simulink model "phase_shift_frequency_control"  (R2018a)
settings: Solver=FixedStepDiscrete  StartTime=0.0  StopTime=stopTime  FixedStep=sampleTime  RelTol=1e-3
InitFcn:
  | fs=160e3; %Hz
  | stopTime=0.01;
  | sampleTime=1e-8;
  | deadtime= round(((1/fs)/20)/sampleTime);
  | Vdc=100;
  | Lp=82e-6;
  | Cp=1/ (Lp*4*pi*pi*150e3*150e3);
  | Rp=0.3;
  | RLOAD=10
libraries: powerlib x10
settings Model: Creator=enes_  LastModifiedBy=enes_

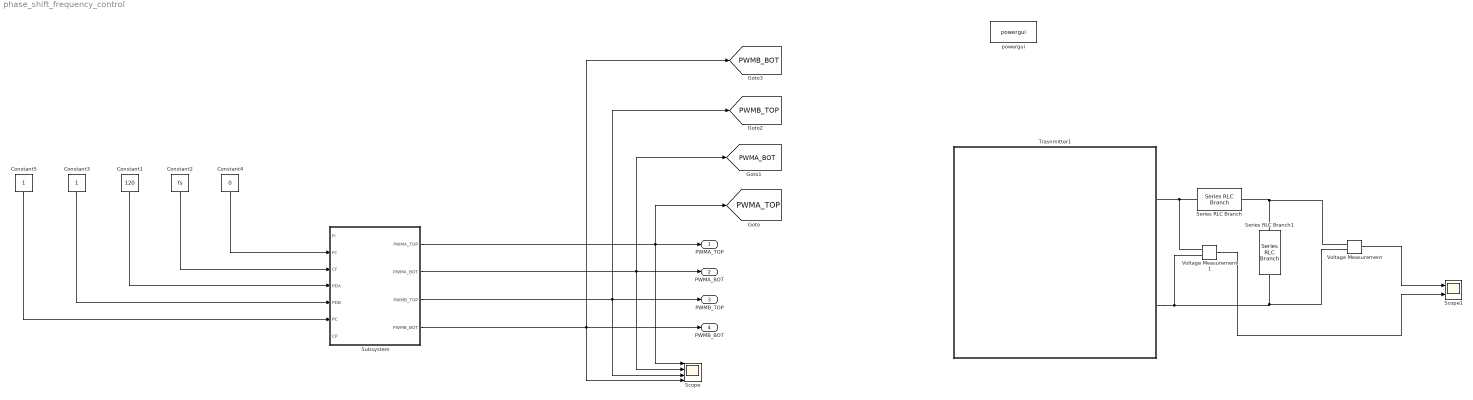
== system phase_shift_frequency_control ==
  Constant1 : Constant  Value=120
  Constant2 : Constant  Value=fs
  Constant3 : Constant
  Constant4 : Constant  Value=0
  Constant5 : Constant
  Scope : Scope  NumInputPorts=4
  Scope1 : Scope  NumInputPorts=2
  Series RLC Branch : powerlib/Elements/Series RLC Branch  LConnTagsString=__new0  RConnTagsString=__new0  BranchType=RLC  Resistance=Rp  Inductance=Lp  SetiL0=off  InitialCurrent=0  Capacitance=Cp  Setx0=off  InitialVoltage=0  Measurements=None
  Series RLC Branch1 : powerlib/Elements/Series RLC Branch  LConnTagsString=__new0  RConnTagsString=__new0  BranchType=R  Resistance=RLOAD  Inductance=Lp  SetiL0=off  InitialCurrent=0  Capacitance=Cp  Setx0=off  InitialVoltage=0  Measurements=None
  Subsystem : Subsystem
  Trasnmitter1 : Subsystem
  Voltage Measurement : powerlib/Measurements/Voltage Measurement  PhasorSimulation=off  OutputType=Complex  PSBequivalent=0
  Voltage Measurement1 : powerlib/Measurements/Voltage Measurement  PhasorSimulation=off  OutputType=Complex  PSBequivalent=0
  powergui : powerlib/powergui  Priority=1  SimulationMode=Discrete  SampleTime=sampleTime  frequency=60  Iterations=50  frequencyindice=0  Pbase=100e6  ErrMax=1e-4  UnitsV=kV  UnitsW=MW  buscounter=0  FunctionMessages=off  echomessages=off  EnableUseOfTLC=off  CurrentSourceSwitches=off  DisableSnubberDevices=off  DisableRonSwitches=off  DisableVfSwitches=off  DisplayEquations=off  SolverType=Tustin/Backward Euler (TBE)  Interpol=off  ExternalGateDelay=off  methode=off  Ts=100  x0status=blocks  SPID=on  SwTol=0  HookPort=off  RestoreLinks=warning  ResistiveCurrentMeasurement=off  Frange=[0:2:500]  Ylog=off  Xlog=on  ShowGrid=off  save=off  variable=ZData  structure=0  ZoomFFT=off  StartTime=0.0  cycles=1  DisplayStyle=1  fundamental=60  FreqAxis=off  MaxFrequency=1000  frequencyindicesteady=1  RmsSteady=1  display=off
  PWMA_TOP : Outport
  PWMA_BOT : Outport  Port=2
  PWMB_TOP : Outport  Port=3
  PWMB_BOT : Outport  Port=4
  tag scope: PWMA_BOT=global, PWMA_TOP=global, PWMB_BOT=global, PWMB_TOP=global
  wires:
  Constant4/1 -> Subsystem/2(FC)
  Constant2/1 -> Subsystem/3(CF)
  Constant1/1 -> Subsystem/4(PDA)
  Constant3/1 -> Subsystem/5(PDB)
  Constant5/1 -> Subsystem/6(PC)
  Subsystem/2(PWMA_BOT) -> [PWMA_BOT], PWMA_BOT/1, Scope/2
  Subsystem/3(PWMB_TOP) -> [PWMB_TOP], Scope/3, PWMB_TOP/1
  Subsystem/4(PWMB_BOT) -> [PWMB_BOT], Scope/4, PWMB_BOT/1
  Subsystem/1(PWMA_TOP) -> [PWMA_TOP], Scope/1, PWMA_TOP/1
  Voltage Measurement/1 -> Scope1/1
  Voltage Measurement1/1 -> Scope1/2
  connections:
  Series RLC Branch/LConn1 -- Voltage Measurement1/LConn1 -- Trasnmitter1/LConn1
  Trasnmitter1/LConn2 -- Voltage Measurement1/LConn2 -- Voltage Measurement/LConn2 -- Series RLC Branch1/RConn1
  Series RLC Branch1/LConn1 -- Voltage Measurement/LConn1 -- Series RLC Branch/RConn1

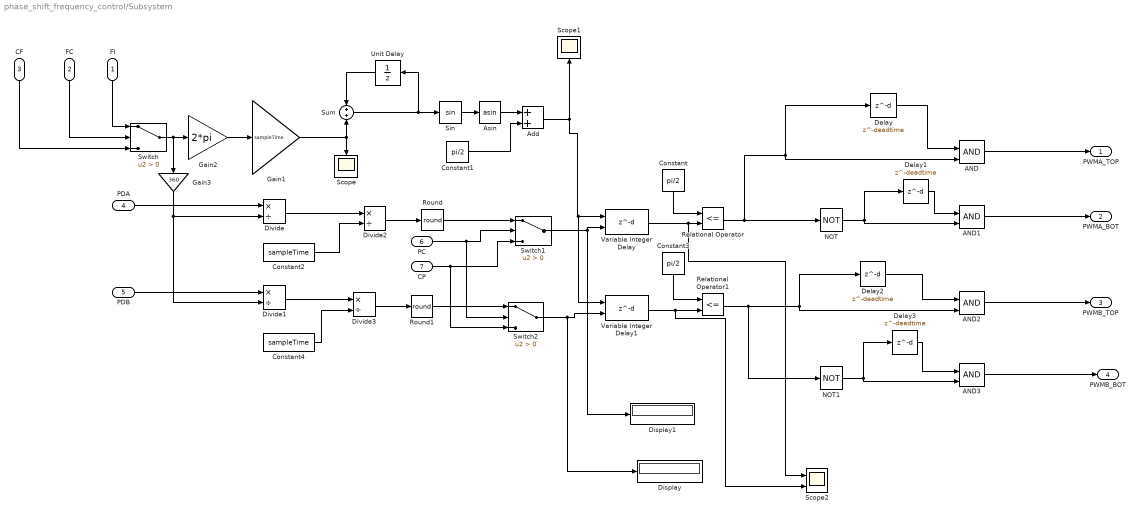
== system phase_shift_frequency_control/Subsystem ==
  FI : Inport
  FC : Inport  Port=2
  CF : Inport  Port=3
  PDA : Inport  Port=4
  PDB : Inport  Port=5
  PC : Inport  Port=6
  CP : Inport  Port=7
  AND{,1..3} (4 alike) : Logic  IconShape=distinctive  AllPortsSameDT=off  OutDataTypeStr=boolean
  Add : Sum
  Asin : Trigonometry  Operator=asin
  Constant : Constant  Value=pi/2
  Constant1 : Constant  Value=pi/2
  Constant2 : Constant  Value=sampleTime
  Constant3 : Constant  Value=pi/2
  Constant4 : Constant  Value=sampleTime
  Delay{,1..3} (4 alike) : Delay  DelayLength=deadtime
  Display : Display
  Display1 : Display
  Divide{,1..3} (4 alike) : Product  Inputs=*/
  Gain1 : Gain  Gain=sampleTime
  Gain2 : Gain  Gain=2*pi
  Gain3 : Gain  Gain=360
  NOT : Logic  Operator=NOT  IconShape=distinctive  AllPortsSameDT=off  OutDataTypeStr=boolean
  NOT1 : Logic  Operator=NOT  IconShape=distinctive  AllPortsSameDT=off  OutDataTypeStr=boolean
  Relational Operator : RelationalOperator  Operator=<=  OutDataTypeStr=boolean  RndMeth=Simplest
  Relational Operator1 : RelationalOperator  Operator=<=  OutDataTypeStr=boolean  RndMeth=Simplest
  Round : Rounding  Operator=round
  Round1 : Rounding  Operator=round
  Scope : Scope
  Scope1 : Scope
  Scope2 : Scope  NumInputPorts=2
  Sin : Trigonometry
  Sum : Sum
  Switch : Switch  Criteria=u2 > Threshold
  Switch1 : Switch  Criteria=u2 > Threshold
  Switch2 : Switch  Criteria=u2 > Threshold
  Unit Delay : UnitDelay  SampleTime=-1
  Variable Integer Delay : Delay  DelayLengthSource=Input port
      settings: InputPortMap=u0,p1
  Variable Integer Delay1 : Delay  DelayLengthSource=Input port
      settings: InputPortMap=u0,p1
  PWMA_TOP : Outport
  PWMA_BOT : Outport  Port=2
  PWMB_TOP : Outport  Port=3
  PWMB_BOT : Outport  Port=4
  wires:
  Gain1/1 -> Sum/2, Scope/1
  AND/1 -> PWMA_TOP/1
  Asin/1 -> Add/1
  CP/1 -> Switch2/3, Switch1/3
  Sum/1 -> Sin/1, Unit Delay/1
  Switch1/1 -> Variable Integer Delay/2, Display1/1
  Gain2/1 -> Gain1/1
  Unit Delay/1 -> Sum/1
  FI/1 -> Switch/1
  CF/1 -> Switch/3
  Constant3/1 -> Relational Operator1/1
  Variable Integer Delay1/1 -> Scope2/2, Relational Operator1/2
  PC/1 -> Switch2/2, Switch1/2
  Constant/1 -> Relational Operator/1
  PDA/1 -> Divide/1
  Relational Operator/1 -> Delay/1, AND/2, NOT/1
  PDB/1 -> Divide1/1
  Gain3/1 -> Divide1/2, Divide/2
  AND2/1 -> PWMB_TOP/1
  Switch/1 -> Gain2/1, Gain3/1
  Switch2/1 -> Display/1, Variable Integer Delay1/2
  FC/1 -> Switch/2
  AND3/1 -> PWMB_BOT/1
  NOT1/1 -> Delay3/1, AND3/2
  Divide/1 -> Divide2/1
  Constant2/1 -> Divide2/2
  Divide2/1 -> Round/1
  Divide3/1 -> Round1/1
  Divide1/1 -> Divide3/1
  Constant4/1 -> Divide3/2
  Variable Integer Delay/1 -> Scope2/1, Relational Operator/2
  Round/1 -> Switch1/1
  Round1/1 -> Switch2/1
  NOT/1 -> Delay1/1, AND1/2
  AND1/1 -> PWMA_BOT/1
  Delay/1 -> AND/1
  Delay1/1 -> AND1/1
  Relational Operator1/1 -> Delay2/1, AND2/2, NOT1/1
  Delay2/1 -> AND2/1
  Delay3/1 -> AND3/1
  Sin/1 -> Asin/1
  Add/1 -> Variable Integer Delay/1, Variable Integer Delay1/1, Scope1/1
  Constant1/1 -> Add/2

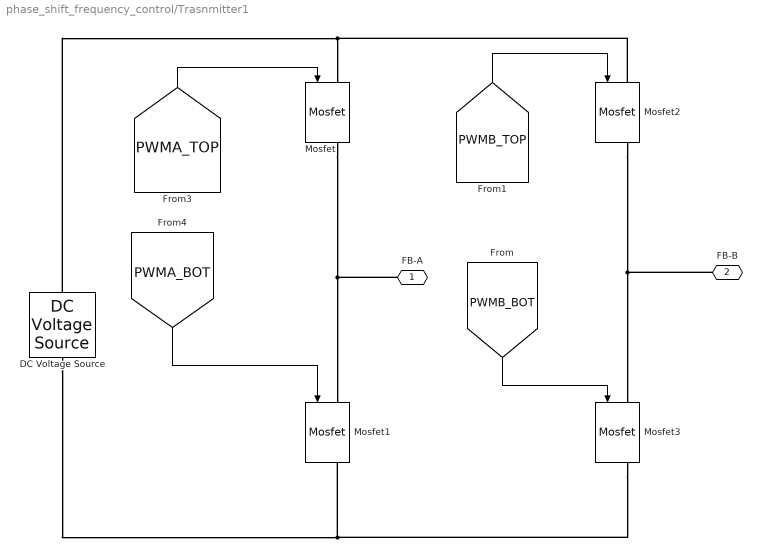
== system phase_shift_frequency_control/Trasnmitter1 ==
  DC Voltage Source : powerlib/Electrical Sources/DC Voltage Source  Amplitude=Vdc  Measurements=None
  Mosfet{,1..3} (4 alike) : powerlib/Power Electronics/Mosfet  Ron=0.1  Lon=0  Rd=0.01  Vfd=0  IC=0  Rs=1e5  Cs=inf  Measurements=on
  FB-A : PMIOPort  Side=Left
  FB-B : PMIOPort  Port=2  Side=Left
  wires:
  [PWMA_TOP] -> Mosfet/1
  [PWMB_BOT] -> Mosfet3/1
  [PWMA_BOT] -> Mosfet1/1
  [PWMB_TOP] -> Mosfet2/1
  connections:
  Mosfet2/RConn1 -- FB-B/RConn1 -- Mosfet3/LConn1
  Mosfet/RConn1 -- FB-A/RConn1 -- Mosfet1/LConn1
  DC Voltage Source/RConn1 -- Mosfet2/LConn1 -- Mosfet/LConn1
  DC Voltage Source/LConn1 -- Mosfet3/RConn1 -- Mosfet1/RConn1
